simulink model "youhua_1226"  (R2017b)
settings: Solver=ode1  StartTime=0.0  StopTime=Inf  FixedStep=0.0002  RelTol=1e-3
PreLoadFcn:
  | initFun_4P.m
PostLoadFcn:
  | , if any(exist('dsrtsu_mdlpostloadfcn', 'file') == [2, 3, 6]), try dsrtsu_mdlpostloadfcn('Execute', bdroot); catch fprintf('Error in PostLoadFcn (dsrtsu_mdlpostloadfcn) for model "%s":\n %s\n', bdroot, lasterr); end, end,
InitFcn:
  | initFun_4P
undefined symbols (not defined in the file): CMAES_B_initial, CMAES_C_initial, CMAES_chiN_initial, CMAES_counteval_initial, CMAES_D_initial, CMAES_eigeneval_initial, CMAES_invsqrtC_initial, CMAES_pc_initial, CMAES_ps_initial, CMAES_sigma_initial, CMAES_xmean_initial
libraries: rti1202lib_adc_class1 x20, simulink x8, dsparch4 x6, rti1202serlib x4, rti1202lib_dio_class1 x4, dsextras x3, rtiemclib x2, rti1202lib_dac_class1 x1, rtitasklib x1
(part 4 of 6)

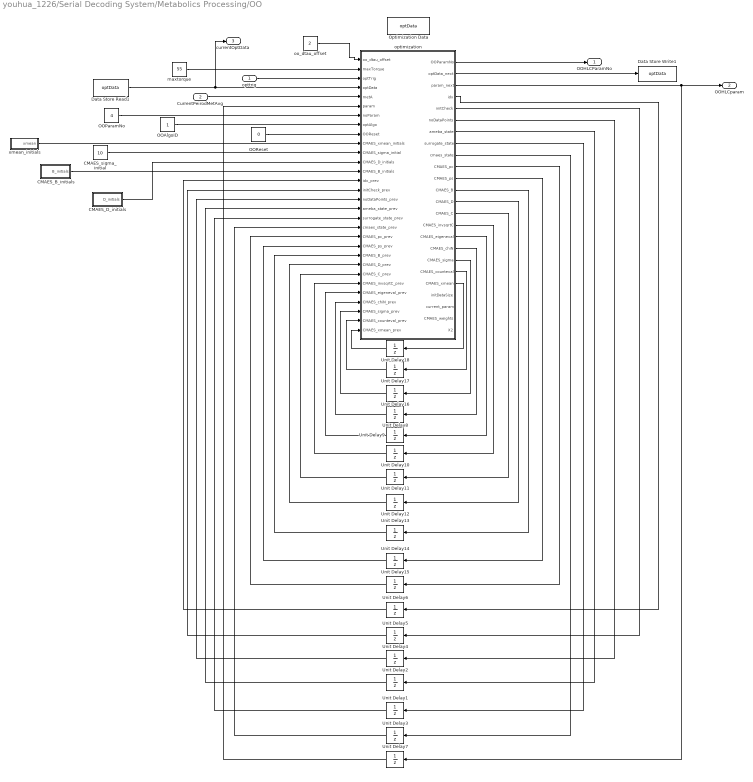
== system youhua_1226/Serial Decoding System/Metabolics Processing/OO ==
  opttrig : Inport
  CurrentPeirodMetAvg : Inport  Port=2
  CMAES_B_initials : Subsystem
  CMAES_D_initials : Subsystem
  CMAES_sigma_initial : Constant  Value=10
  Data Store Read1 : DataStoreRead  DataStoreName=optData
  Data Store Write1 : DataStoreWrite  DataStoreName=optData
  OOAlgoID : Constant
  OOParamNo : Constant  Value=4
  OOReset : Constant  Value=0
  Optimization Data : DataStoreMemory  DataStoreName=optData  ReadBeforeWriteMsg=warning  WriteAfterWriteMsg=warning  WriteAfterReadMsg=warning  InitialValue=zeros(8,5)  ShowAdditionalParam=off
  Unit Delay{1..6} (6 alike) : UnitDelay  SampleTime=-1
  Unit Delay10 : UnitDelay  InitialCondition=CMAES_invsqrtC_initial  SampleTime=-1
  Unit Delay11 : UnitDelay  InitialCondition=CMAES_C_initial  SampleTime=-1
  Unit Delay12 : UnitDelay  InitialCondition=CMAES_D_initial  SampleTime=-1
  Unit Delay13 : UnitDelay  InitialCondition=CMAES_B_initial  SampleTime=-1
  Unit Delay14 : UnitDelay  InitialCondition=CMAES_ps_initial  SampleTime=-1
  Unit Delay15 : UnitDelay  InitialCondition=CMAES_pc_initial  SampleTime=-1
  Unit Delay16 : UnitDelay  InitialCondition=CMAES_sigma_initial  SampleTime=-1
  Unit Delay17 : UnitDelay  InitialCondition=CMAES_counteval_initial  SampleTime=-1
  Unit Delay18 : UnitDelay  InitialCondition=CMAES_xmean_initial  SampleTime=-1
  Unit Delay7 : UnitDelay  InitialCondition=zeros(4,1)  SampleTime=-1
  Unit Delay8 : UnitDelay  InitialCondition=CMAES_chiN_initial  SampleTime=-1
  Unit Delay9 : UnitDelay  InitialCondition=CMAES_eigeneval_initial  SampleTime=-1
  maxtorque : Constant  Value=55
  oo_dtau_offset : Constant  Value=2
  optimization : MATLAB Function  TreatAsAtomicUnit=on
  xmean_initials : Subsystem
  OOHLCParamNo : Outport
  OOHLCparam : Outport  Port=2
  currentOptData : Outport  Port=3
  wires:
  Data Store Read1/1 -> optimization/4(optData), currentOptData/1
  OOAlgoID/1 -> optimization/8(optAlgo)
  CurrentPeirodMetAvg/1 -> optimization/5(metA)
  optimization/3(param_next) -> Unit Delay7/1, OOHLCparam/1
  optimization/2(optData_next) -> Data Store Write1/1
  optimization/1(OOParamNo) -> OOHLCParamNo/1
  OOParamNo/1 -> optimization/7(noParam)
  optimization/4(idx) -> Unit Delay6/1
  Unit Delay7/1 -> optimization/6(param)
  Unit Delay6/1 -> optimization/14(idx_prev)
  OOReset/1 -> optimization/9(OOReset)
  optimization/5(initCheck) -> Unit Delay5/1
  Unit Delay5/1 -> optimization/15(initCheck_prev)
  optimization/6(noDataPoints) -> Unit Delay4/1
  Unit Delay4/1 -> optimization/16(noDataPoints_prev)
  Unit Delay2/1 -> optimization/17(ameba_state_prev)
  optimization/7(ameba_state) -> Unit Delay2/1
  optimization/8(surrogate_state) -> Unit Delay1/1
  Unit Delay1/1 -> optimization/18(surrogate_state_prev)
  optimization/9(cmaes_state) -> Unit Delay3/1
  Unit Delay3/1 -> optimization/19(cmaes_state_prev)
  optimization/17(CMAES_chiN) -> Unit Delay8/1
  Unit Delay8/1 -> optimization/27(CMAES_chiN_prev)
  optimization/16(CMAES_eigeneval) -> Unit Delay9/1
  Unit Delay9/1 -> optimization/26(CMAES_eigeneval_prev)
  optimization/15(CMAES_invsqrtC) -> Unit Delay10/1
  Unit Delay10/1 -> optimization/25(CMAES_invsqrtC_prev)
  optimization/14(CMAES_C) -> Unit Delay11/1
  Unit Delay11/1 -> optimization/24(CMAES_C_prev)
  optimization/13(CMAES_D) -> Unit Delay12/1
  optimization/12(CMAES_B) -> Unit Delay13/1
  optimization/11(CMAES_ps) -> Unit Delay14/1
  optimization/10(CMAES_pc) -> Unit Delay15/1
  Unit Delay12/1 -> optimization/23(CMAES_D_prev)
  Unit Delay13/1 -> optimization/22(CMAES_B_prev)
  Unit Delay14/1 -> optimization/21(CMAES_ps_prev)
  Unit Delay15/1 -> optimization/20(CMAES_pc_prev)
  optimization/18(CMAES_sigma) -> Unit Delay16/1
  Unit Delay16/1 -> optimization/28(CMAES_sigma_prev)
  optimization/19(CMAES_counteval) -> Unit Delay17/1
  Unit Delay17/1 -> optimization/29(CMAES_counteval_prev)
  optimization/20(CMAES_xmean) -> Unit Delay18/1
  Unit Delay18/1 -> optimization/30(CMAES_xmean_prev)
  opttrig/1 -> optimization/3(optTrig)
  CMAES_sigma_initial/1 -> optimization/11(CMAES_sigma_initial)
  xmean_initials/1(xmean) -> optimization/10(CMAES_xmean_initials)
  CMAES_D_initials/1(D_initials) -> optimization/12(CMAES_D_initials)
  maxtorque/1 -> optimization/2(maxTorque)
  CMAES_B_initials/1(B_initials) -> optimization/13(CMAES_B_initials)
  oo_dtau_offset/1 -> optimization/1(oo_dtau_offset)

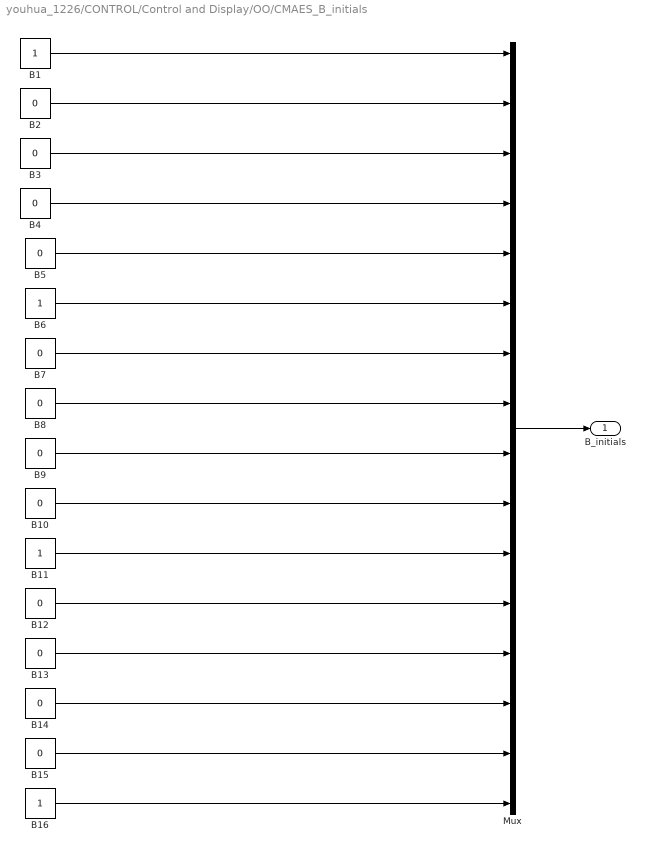
== system youhua_1226/CONTROL/Control and Display/OO/CMAES_B_initials ==
  B{1,6,11,16} (4 alike) : Constant
  B{2..5,7..10,12..15} (12 alike) : Constant  Value=0
  Mux : Mux  Inputs=16
  B_initials : Outport
  wires:
  B1/1 -> Mux/1
  B3/1 -> Mux/3
  B4/1 -> Mux/4
  B2/1 -> Mux/2
  Mux/1 -> B_initials/1
  B5/1 -> Mux/5
  B7/1 -> Mux/7
  B8/1 -> Mux/8
  B6/1 -> Mux/6
  B9/1 -> Mux/9
  B11/1 -> Mux/11
  B12/1 -> Mux/12
  B10/1 -> Mux/10
  B13/1 -> Mux/13
  B15/1 -> Mux/15
  B16/1 -> Mux/16
  B14/1 -> Mux/14

== system youhua_1226/CONTROL/Control and Display/OO/CMAES_D_initials ==
  D{1..4} (4 alike) : Constant
  Mux : Mux
  D_initials : Outport
  wires:
  D1/1 -> Mux/1
  D3/1 -> Mux/3
  D4/1 -> Mux/4
  D2/1 -> Mux/2
  Mux/1 -> D_initials/1

== system youhua_1226/CONTROL/Control and Display/OO/xmean_initials ==
  Mux : Mux
  xmean1 : Constant  Value=25
  xmean2 : Constant  Value=90
  xmean3 : Constant  Value=25
  xmean4 : Constant  Value=20
  xmean : Outport
  wires:
  xmean1/1 -> Mux/1
  xmean3/1 -> Mux/3
  xmean4/1 -> Mux/4
  xmean2/1 -> Mux/2
  Mux/1 -> xmean/1

== system youhua_1226/CONTROL/Control and Display/learning data read/filtered step data read ==
  indices : Inport
  comm delay cycle : Inport  Port=2
  learningMode : Inport  Port=3
  "   " : SignalSpecification  Dimensions=3
  "       currentstepdata" : DataStoreRead  DataStoreName=filteredStepData
  Step Data Access : MATLAB Function  TreatAsAtomicUnit=on
  oldD : Outport
  wires:
  "       currentstepdata"/1 -> Step Data Access/2(oldSD)
  Step Data Access/1(oldD) -> "   "/1
  indices/1 -> Step Data Access/1(indices)
  "   "/1 -> oldD/1
  comm delay cycle/1 -> Step Data Access/3(CommDelayCycle)
  learningMode/1 -> Step Data Access/4(learningMode)

== system youhua_1226/CONTROL/Control and Display/learning data write/filtered step data write ==
  indices : Inport
  filteredstepdata : Inport  Port=2
  learningMode : Inport  Port=3
  BT Reset3 : Constant  Value=0
  MATLAB Function2 : MATLAB Function  TreatAsAtomicUnit=on
  filtered data store read : DataStoreRead  DataStoreName=filteredStepData
  filtered data store write : DataStoreWrite  DataStoreName=filteredStepData
  wires:
  filtered data store read/1 -> MATLAB Function2/4(filtered_step_data_in)
  MATLAB Function2/1(filtered_step_data_out) -> filtered data store write/1
  BT Reset3/1 -> MATLAB Function2/1(bt_reset3)
  indices/1 -> MATLAB Function2/2(indices)
  filteredstepdata/1 -> MATLAB Function2/3(filtered_step_data)
  learningMode/1 -> MATLAB Function2/5(learningMode)

== system youhua_1226/CONTROL/Control and Display/time derivatives /get ddot torque ==
  data : Inport
  Butterworth Filter (low 100Hz) : DiscreteFilter  Numerator="[0.0181    0.0543    0.0543    0.0181]"  Denominator="[ 1.0000   -1.7600    1.1829   -0.2781]"
  Discrete Derivative : simulink/Discrete/Discrete Derivative  gainval=1.0  ICPrevScaledInput=0.0  InputProcessing=Inherited  OutMin=[]  OutMax=[]  OutDataType=fixdt(1, 16)  OutScaling=2^-10  DoSatur=off
  dotdata : Outport
  wires:
  Discrete Derivative/1 -> Butterworth Filter (low 100Hz)/1
  data/1 -> Discrete Derivative/1
  Butterworth Filter (low 100Hz)/1 -> dotdata/1

== system youhua_1226/CONTROL/Control and Display/time derivatives /get desired torque  ==
  data : Inport
  Butterworth Filter (low 100Hz) : DiscreteFilter  Numerator="[0.0181    0.0543    0.0543    0.0181]"  Denominator="[ 1.0000   -1.7600    1.1829   -0.2781]"
  Discrete Derivative : simulink/Discrete/Discrete Derivative  gainval=1.0  ICPrevScaledInput=0.0  InputProcessing=Inherited  OutMin=[]  OutMax=[]  OutDataType=fixdt(1, 16)  OutScaling=2^-10  DoSatur=off
  dotdata : Outport
  wires:
  Discrete Derivative/1 -> Butterworth Filter (low 100Hz)/1
  data/1 -> Discrete Derivative/1
  Butterworth Filter (low 100Hz)/1 -> dotdata/1

== system youhua_1226/CONTROL/Control and Display/time derivatives /get desired torque 1 ==
  data : Inport
  Butterworth Filter (low 100Hz) : DiscreteFilter  Numerator="[0.0181    0.0543    0.0543    0.0181]"  Denominator="[ 1.0000   -1.7600    1.1829   -0.2781]"
  Discrete Derivative : simulink/Discrete/Discrete Derivative  gainval=1.0  ICPrevScaledInput=0.0  InputProcessing=Inherited  OutMin=[]  OutMax=[]  OutDataType=fixdt(1, 16)  OutScaling=2^-10  DoSatur=off
  dotdata : Outport
  wires:
  Discrete Derivative/1 -> Butterworth Filter (low 100Hz)/1
  data/1 -> Discrete Derivative/1
  Butterworth Filter (low 100Hz)/1 -> dotdata/1

== system youhua_1226/CONTROL/Control and Display/time derivatives /get desired torque 2 ==
  data : Inport
  Butterworth Filter (low 100Hz) : DiscreteFilter  Numerator="[0.0181    0.0543    0.0543    0.0181]"  Denominator="[ 1.0000   -1.7600    1.1829   -0.2781]"
  Discrete Derivative : simulink/Discrete/Discrete Derivative  gainval=1.0  ICPrevScaledInput=0.0  InputProcessing=Inherited  OutMin=[]  OutMax=[]  OutDataType=fixdt(1, 16)  OutScaling=2^-10  DoSatur=off
  dotdata : Outport
  wires:
  Discrete Derivative/1 -> Butterworth Filter (low 100Hz)/1
  data/1 -> Discrete Derivative/1
  Butterworth Filter (low 100Hz)/1 -> dotdata/1

== system youhua_1226/RTI Data/RTI Data Store/RTI Data Store/RTI Data Store ==
  RTI Data Store : Subsystem  mask(RTI_DATA_STORE){}
      mask help:
      | RTI Data Store Block. This block is used by RTI to store internal model dependent data. Deleting this block will result in data loss.
      |
      | NEVER DELETE, COPY, OR MODIFY THIS BLOCK!
      mask Help:
      | RTI Data Store Block. This block is used by RTI to store internal model dependent data. Deleting this block will result in data loss.
      | 
      | NEVER DELETE, COPY, OR MODIFY THIS BLOCK!
      mask Display: text(0.5, 0.5, ' ', 'HorizontalAlignment', 'center');

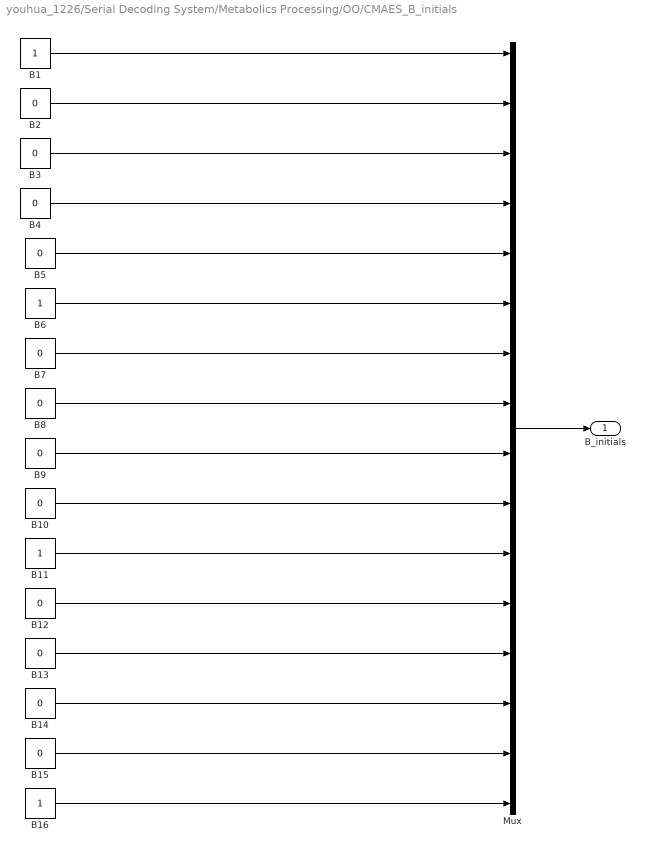
== system youhua_1226/Serial Decoding System/Metabolics Processing/OO/CMAES_B_initials ==
  B{1,6,11,16} (4 alike) : Constant
  B{2..5,7..10,12..15} (12 alike) : Constant  Value=0
  Mux : Mux  Inputs=16
  B_initials : Outport
  wires:
  B1/1 -> Mux/1
  B3/1 -> Mux/3
  B4/1 -> Mux/4
  B2/1 -> Mux/2
  Mux/1 -> B_initials/1
  B5/1 -> Mux/5
  B7/1 -> Mux/7
  B8/1 -> Mux/8
  B6/1 -> Mux/6
  B9/1 -> Mux/9
  B11/1 -> Mux/11
  B12/1 -> Mux/12
  B10/1 -> Mux/10
  B13/1 -> Mux/13
  B15/1 -> Mux/15
  B16/1 -> Mux/16
  B14/1 -> Mux/14

== system youhua_1226/Serial Decoding System/Metabolics Processing/OO/CMAES_D_initials ==
  D{1..4} (4 alike) : Constant
  Mux : Mux
  D_initials : Outport
  wires:
  D1/1 -> Mux/1
  D3/1 -> Mux/3
  D4/1 -> Mux/4
  D2/1 -> Mux/2
  Mux/1 -> D_initials/1

== system youhua_1226/Serial Decoding System/Metabolics Processing/OO/xmean_initials ==
  Mux : Mux
  xmean1 : Constant  Value=25
  xmean2 : Constant  Value=90
  xmean3 : Constant  Value=25
  xmean4 : Constant  Value=20
  xmean : Outport
  wires:
  xmean1/1 -> Mux/1
  xmean3/1 -> Mux/3
  xmean4/1 -> Mux/4
  xmean2/1 -> Mux/2
  Mux/1 -> xmean/1

== system youhua_1226/RTI Data/RTI Data Store/RTI Data Store/RTI Data Store/RTI Data Store ==

== matlab function youhua_1226/Sensor Data Conversion/bit data processing ==
  data: bit_data input; heel_switch output
function heel_switch = fcn(bit_data)

heel_switch = bit_data(1);

% heel_switch = ~heel_switch;

return;

== matlab function youhua_1226/Sensor Data Conversion/analog data processing ==
  data: adc_data input; ankle_pos output; enc_pos input; load_vol_gain input; load_vol_offset input; CPR_ankle input; CPR_motor input; analog_enc_max input; analog_enc_min input; BT_RESET_TORQUE input; force_input0_prev input; motor_pos output; load_cell_vol output; force_input output; EMG1_vol output; force_input0_next output; fzright_raw output; fzleft_raw output
function [ankle_pos, motor_pos, load_cell_vol, force_input, EMG1_vol, force_input0_next,...
    fzright_raw, fzleft_raw]=fcn(adc_data,enc_pos,...
    load_vol_gain,load_vol_offset, CPR_ankle, CPR_motor, analog_enc_max,...
    analog_enc_min, BT_RESET_TORQUE, force_input0_prev)
%#eml
ankle_pos = enc_pos(1)*360/CPR_ankle;
%% analog encoder
% ankle_pos = (adc_data(17)-analog_enc_min)*360/(analog_enc_max-analog_enc_min);
% if ankle_pos >180
%     ankle_pos = ankle_pos - 360;
% end;
% ankle_pos = - ankle_pos;
%%
motor_pos = enc_pos(2)*360/CPR_motor;%CPR_motor = 1250光栅参数
%load_cell_vol 放大器输出电压*10的数值
load_cell_vol = adc_data(6);
%电压力矩转换 load_vol_gain = 9.9206 load_vol_offset = 11.4484；
%force_input_raw  =   load_cell_vol*load_vol_gain/5.5 + load_vol_offset;
force_input_raw  =   load_cell_vol*load_vol_gain + load_vol_offset;
% force_input_raw = max(force_input_raw, 0);
% 力矩调零 BT_RESET_TORQUE （力矩调零按钮）
if BT_RESET_TORQUE ==1
    force_input0_next = force_input_raw;
    
else
    force_input0_next = force_input0_prev;
    
end

force_input = force_input_raw - force_input0_next;
%未知
EMG1_vol = adc_data(5);

fzright_raw = adc_data(11);
fzleft_raw = adc_data(15);

return

== matlab function youhua_1226/CONTROL/Control and Display/State Operation ==
  data: tmp1 output; tmp2 output; reset_torque_swing input; max_desired_torque input; max_motor_pos input; max_motor_pos_inv input; desired_motor_velocity output; current_state_input input; analog_inputs input; user_inputs input; digital_inputs input; state_variables0 input; time input; time_derivatives input; filtered_lrn_data input; CusHLCInputs input; serial_data input; opt_data input; desired_vel_prev input; tau_offset_prev input; state_variables output; current_step_data output; Params output; measured_torque output; ankle_pos output; motor_pos output; desired_torque output; tau_offset output
function [tmp1, tmp2, desired_motor_velocity, state_variables, current_step_data,Params,measured_torque,ankle_pos,motor_pos,desired_torque, tau_offset]  =...
    fcn(reset_torque_swing, max_desired_torque,max_motor_pos,max_motor_pos_inv,current_state_input, analog_inputs,user_inputs, digital_inputs,...
    state_variables0, time,  time_derivatives, filtered_lrn_data,...
    CusHLCInputs,serial_data, opt_data, desired_vel_prev,tau_offset_prev)


% defination
%State definitions
idle_state	=	0;
calibration_state	=   1;
stance_state   =   2;
swing_state     =   3;
step_state  =   4;
slack_state = 5;
pos_track_state = 6;
%   Constants
gearRatio = 5;



maximum_motor_velocity = 90*360; %maximum allowable motor velocity (deg/s)


current_state = current_state_input(1);
stop_pos = current_state_input(2);
slack_pos = current_state_input(3);
stance_end_pos = current_state_input(4);
flag_d_p = current_state_input(6);
dorsi_end_pos = current_state_input(15);
last_stride_time = current_state_input(13);


% vo2 = serial_data(1);
% vco2 = serial_data(2);
% metE = serial_data(3);
%
% metA = opt_data(1);
HLCParamNo = opt_data(2);
HLCParam = opt_data(3:HLCParamNo+2);
Params = opt_data(3:end);



% load_pivot_distance = 0;
% load_angle = 0;

% state variables initialization
zero_ankle_pos_prev =  state_variables0(1);
zero_motor_pos_prev = state_variables0(2);
ankle_pos_prev = state_variables0(3);
motor_pos_prev = state_variables0(4);
desired_torque_prev = state_variables0(5);
measured_torque_prev = state_variables0(6);
measured_force_prev = state_variables0(7);
load_angle_prev = state_variables0(8);
load_pivot_distance_prev = state_variables0(9);
delta_motor_pos_prev = state_variables0(10);
slack_motor_pos_prev = state_variables0(11);
torque_error_prev = state_variables0(12);
Kp_prev = state_variables0(13);
ankle_vel_prev = state_variables0(14);
motor_vel_prev = state_variables0(15);
motor_acc_prev = state_variables0(16);
Kd_prev = state_variables0(17);
Ki_prev = state_variables0(18);
Controller_prev = state_variables0(19);
Kc_prev = state_variables0(20);
time_prev = state_variables0(21);
state_prev = state_variables0(22);
state_start_time_prev = state_variables0(23);
curve_id_prev = state_variables0(24);
Kpp_prev = state_variables0(25);
accumulated_torque_error_prev = state_variables0(26);
desired_motor_pos_prev = state_variables0(27);
walk_control_mode_prev = state_variables0(28);
prev_step_accumulated_error_prev = state_variables0(29);
curr_step_accumulated_error_prev = state_variables0(30);
learning_control_input_prev = state_variables0(31);

learning_control_input2_prev = state_variables0(32);
Kp2_prev = state_variables0(33);
Kl_prev = state_variables0(34);
Kl2_prev = state_variables0(35);
gamma_prev = state_variables0(37);
Lce_prev = state_variables0(38);
Lmtu_prev = state_variables0(39);
FL_prev = state_variables0(40);
Fpe_prev = state_variables0(41);
ACT_prev = state_variables0(42);
STIM_Prev = state_variables0(43);
Fmtu_prev = state_variables0(44);
Lcedot_prev = state_variables0(45);
learned_value_prev = state_variables0(46);
learned_avg_prev = state_variables0(47);
accumulated_pos_error_prev = state_variables0(48);
gamma1_prev = state_variables0(49);
gamma2_prev = state_variables0(50);
gamma3_prev = state_variables0(51);
gamma4_prev = state_variables0(52);
gamma_v_prev = [gamma1_prev;gamma2_prev;gamma3_prev;gamma4_prev];




%% if no updation, use the old ones
zero_motor_pos = zero_motor_pos_prev; %if no new zero points set, keep old ones
zero_ankle_pos = zero_ankle_pos_prev;
ankle_pos = ankle_pos_prev;
motor_pos = motor_pos_prev;
desired_torque = desired_torque_prev;
measured_torque = measured_torque_prev;
measured_force = measured_force_prev;
load_angle = load_angle_prev;
load_pivot_distance = load_pivot_distance_prev;
delta_motor_pos = delta_motor_pos_prev;
slack_motor_pos = slack_motor_pos_prev;
torque_error = torque_error_prev;
Kp = Kp_prev;
ankle_vel = ankle_vel_prev;
motor_vel = motor_vel_prev;
motor_acc = motor_acc_prev;
Kd = Kd_prev;
Ki = Ki_prev;
Controller = Controller_prev;
Kc = Kc_prev;
current_time = time_prev;
state = state_prev;
state_start_time = state_start_time_prev;
curve_id = curve_id_prev;
Kpp = Kpp_prev;
accumulated_torque_error = accumulated_torque_error_prev;
desired_motor_pos = desired_motor_pos_prev;
walk_control_mode  = walk_control_mode_prev;
prev_step_accumulated_error=prev_step_accumulated_error_prev;
curr_step_accumulated_error=curr_step_accumulated_error_prev;
learning_control_input = learning_control_input_prev;
learning_control_input2 = learning_control_input2_prev;
Kp2 = Kp2_prev;
Kl = Kl_prev;
Kl2 = Kl2_prev;
gamma = gamma_prev;

Lce = Lce_prev;
Lmtu = Lmtu_prev;
FL = FL_prev;
Fpe = Fpe_prev;
ACT = ACT_prev ;
STIM = STIM_Prev ;
Fmtu = Fmtu_prev ;
Lcedot = Lcedot_prev;
learned_value  = learned_value_prev;
learned_avg = learned_avg_prev;
accumulated_pos_error = accumulated_pos_error_prev;
gamma1 = gamma1_prev;
gamma2 = gamma2_prev;
gamma3 = gamma3_prev;
gamma4 = gamma4_prev;
gamma_v = gamma_v_prev;
state_variables = state_variables0;

% learned_avg = step_avg_data;


tau_offset = tau_offset_prev;







% foot_switch     =   digital_inputs(1);
load_cell_vol = analog_inputs(3);
measured_ankle_pos = analog_inputs(1);
measured_motor_pos = analog_inputs(2);
measured_force = analog_inputs(4);
ankle_vel = analog_inputs(5);
motor_vel = analog_inputs(6);
force_vel = analog_inputs(7);
motor_acc = analog_inputs(8);
EMG1_vol = analog_inputs(9);


Kp = user_inputs(1);
load_distance_1 = user_inputs(2); % in inches
load_distance_2 = user_inputs(3); % in inches
load_ankle_offset = user_inputs(4); % in degrees
delta_t_motor = user_inputs(6);
user_motor_speed = user_inputs(7);
desired_torque = user_inputs(8);
Kd = user_inputs(9);
Ki = user_inputs(10);
Controller = user_inputs(11);
Kc = user_inputs(12);
system_delay = user_inputs(13)/1000;
curve_id = user_inputs(14);
Kpp = user_inputs(15);
sine_freq = user_inputs(16);
Kt = user_inputs(17);
stance_motor_offset = user_inputs(18);
stance_motor_speed = user_inputs(19);
swing_motor_slack = user_inputs(20);
walk_control_mode = user_inputs(21);
slack_length = user_inputs(22);
desired_torque_magnitude = user_inputs(23);
Kl = user_inputs(24);
Kl2 = user_inputs(25);
x1 = user_inputs(26);
y1 = user_inputs(27);
xinit = user_inputs(28);
xturn = user_inputs(29);
yturn = user_inputs(30);
Cw = user_inputs(31);
Kpa= user_inputs(32);
load_pivot_distance = user_inputs(33);
torque_offset = user_inputs(34);
K_curve = user_inputs(35);
K_amp = user_inputs(36);
K_s = user_inputs(37);
L_adpt = user_inputs(38);


%% parameters of NMM

est_stride_time = user_inputs(54);
EMG_OFFSET = user_inputs(58);


%% eroror dependant p parames
ed_p_taumax = user_inputs(60);
ed_p_taustep = user_inputs(61);
%%
comm_delay_cycle = user_inputs(62);
isModiAdded = user_inputs(63);
%% position tracking performance test
Pos_Kd = user_inputs(64);
Pos_Ki = user_inputs(65);
%%
alpha = user_inputs (66);

%% passivity
lambda = user_inputs(67);
%%
isPosPID = user_inputs(68);
%% for learning control threshold

lrn_tau_err_threshold = user_inputs(69);
lrn_shrink_rate = user_inputs(70);

K_swing_follow = user_inputs(72);
r_motor_shaft = user_inputs(73);

%% for ankle-based curve

maxPlanter = user_inputs(74);
xadjust_ref = user_inputs(75);
yadjust_ref = user_inputs(76);


curve_k2 = user_inputs(78);
pos_traj_mode = user_inputs(79);
pos_des_1 = user_inputs(80);
pos_des_2 = user_inputs(81);

Kp_early_swing = user_inputs(82);

oo_dtau_offset = user_inputs(83);


%% for learning control
previous_filtered_torque_error = filtered_lrn_data(1); %torque error of same index of last step

previous_learning_control_input = filtered_lrn_data(2);
predicted_learning_control_input = filtered_lrn_data(3);

% torque_error = previous_filtered_torque_error;
current_learning_control_input = previous_learning_control_input;
current_step_data = [torque_error; current_learning_control_input; previous_filtered_torque_error];

%%
% 脚踝与电机编码器角度调零
motor_pos = measured_motor_pos - zero_motor_pos;
ankle_pos = measured_ankle_pos - zero_ankle_pos;


% load_input      =   load_cell_vol*load_vol_gain + load_vol_offset;
% if measured_force < 0
%     measured_force = 0;
% end;
load_angle = load_ankle_offset - ankle_pos;
% load_pivot_distance = load_distance_1*load_distance_2*sin(load_angle*pi/180)/sqrt(load_distance_1^2+load_distance_2^2+2*load_distance_1*load_distance_2*cos(load_angle*pi/180));
% load_pivot_distance = 3.7808;
% 1`111111111111111`1
% measured_torque =   measured_force*load_pivot_distance-torque_offset;
% 原本是在此处由力转成力矩，由于之前force_input已经直接转化为力矩，所以这里直接用 measured_torque =   measured_force;
% measured_torque = max(0, measured_torque);
measured_torque =   measured_force;


% desired_torque  =   20;

%%%%%%%%%%%%%%%%%%% state variables update%%%%%%%%%%%%%%%%%%%%%%%%%%%%%%%%%
current_time = time;
state = current_state;

%--------------
tmp1 = state;
tmp2 = state_prev;
%--------------
if state~= state_prev
    state_start_time = current_time;
    accumulated_torque_error = 0;
    accumulated_pos_error = 0;
    gamma1_prev = 0;
    gamma2_prev = 0;
    gamma3_prev = 0;
    gamma4_prev = 0;
    if state == stance_state
        prev_step_accumulated_error = curr_step_accumulated_error;
        curr_step_accumulated_error = 0;
        learning_control_input = 0;
        
    end;
    if state == idle_state
        prev_step_accumulated_error = 0;
        curr_step_accumulated_error = 0;
        learning_control_input = 0;
        Kp2 = 0;
        learning_control_input2 =0;
    end;
    if state == swing_state && state_prev ~= stance_state % start of walk
        %         gamma1 = 0;
        %         gamma2 = 0;
        %         gamma3 = 0;
        %         gamma4 = 0;
        %         gamma_v = [0 0 0 0]';
        gamma1_prev = 0;
        gamma2_prev = 0;
        gamma3_prev = 0;
        gamma4_prev = 0;
        %         gamma_v_prev  = [ 0 0 0 0]';
    end
end;

%%%%%%%%%%% variables update finished
if flag_d_p==0
    Cw=0;
end;



%生成期望力矩曲线；curve_id：期望曲线类型  last_stride_time: 1 or 1.5  
%CusHLCInputs 力矩曲线的四参数 ：peak_torque peak_time rise_time drop_time
%oo_dtau_offset
%HLCParam
%xinit
desired_torque = torque_curve(current_time, state_start_time,...
    current_state, curve_id,...
    desired_torque_magnitude,...
    last_stride_time, HLCParam, ankle_pos, xinit,K_curve, CusHLCInputs, oo_dtau_offset);
%期望力矩不能超过120（单位不一样可能需要调整）
desired_torque = min(desired_torque, max_desired_torque);
if state==stance_state
    torque_error = measured_torque-desired_torque;
else
    torque_error = 0;
end

%% for learning with filtered torque
filtered_torque_error = previous_filtered_torque_error*(1-alpha) + alpha*torque_error;
%%
accumulated_torque_error = torque_error + accumulated_torque_error;
accumulated_pos_error = accumulated_pos_error_prev + desired_motor_pos - motor_pos;
if state == stance_state
    curr_step_accumulated_error = curr_step_accumulated_error + torque_error*0.002;
end


%% time derivatives
dot_desired_torque = time_derivatives(1);
ddot_desired_torque = time_derivatives(2);
dot_desired_motor_pos = time_derivatives(3);
dot_measured_torque = time_derivatives(4);

%% passivity based control 存疑
% s = lambda*torque_error + dot_measured_torque-dot_desired_torque;
% Y = [measured_torque; dot_desired_torque-lambda*torque_error; ddot_desired_torque-lambda*(dot_measured_torque - dot_desired_torque); ankle_vel]';
s = lambda*torque_error -motor_vel;
Y = [measured_torque; -lambda*torque_error; lambda*motor_vel; ankle_vel]';
gamma_v_prev = [gamma1_prev;gamma2_prev;gamma3_prev;gamma4_prev];
gamma_v = gamma_v_prev + delta_t_motor*(-L_adpt*Y'*s);
% Y = 0
% gamma_v = [ 0 0 0 0]';
gamma1 = gamma_v(1);
gamma2 = gamma_v(2);
gamma3 = gamma_v(3);
gamma4 = gamma_v(4);


% 存疑 
motor_pos_modifer = isModiAdded*motor_vel*comm_delay_cycle*0.002*gearRatio/delta_t_motor;
posTrack_modifier = isPosPID*(-Pos_Kd*(dot_desired_motor_pos - motor_vel)*gearRatio-Pos_Ki*gearRatio*accumulated_pos_error);


% 力矩调零 由于reset_torque_swing = 0 所以暂时没用到 tau_offset = 0
if reset_torque_swing ==1
    if current_state == swing_state
        if (current_time - state_start_time)> 0.15 && (current_time - state_start_time)< 0.2
            tau_offset = measured_torque;
        end
    end
end

if reset_torque_swing ==2
tau_offset = 0;
end

measured_torque = measured_torque - tau_offset; % dynamic resetting 

switch current_state
    case idle_state
        %               desired_motor_velocity = -(motor_pos-motor_pos_prev)/delta_t_motor;
        if stop_pos == 0 %stop_pos = motor_pos_prev
            desired_motor_velocity = 0;
        else
            delta_motor_pos = (stop_pos -motor_pos);
            desired_motor_pos = stop_pos;
            desired_motor_velocity = -(delta_motor_pos*gearRatio/delta_t_motor);
        end
    % 调整脚踝与电机编码器角度为零的状态，记录当前编码器角度，下一个采样时做差调零
    case calibration_state 
        zero_motor_pos = measured_motor_pos;
        zero_ankle_pos = measured_ankle_pos;
        slack_motor_pos = measured_motor_pos;
        desired_motor_velocity = user_motor_speed;
        %       desired_torque = torque_curve(current_time, state_start_time, Controller, current_state, curve_id, sine_freq, ankle_pos, Kt);
    % 未知    
    case step_state
        switch Controller
            
            otherwise
                desired_motor_velocity = 0;
        end
        
    case stance_state
        %delta_t_motor的值可能需要调整，当前为0.05 会使控制电压过大
        switch walk_control_mode
            case 1 % torque control % PAPER CONTROLLER 1 & 2, Kpp = zero, nonzero 力矩控制 Kpp = 0 Ki = 0
                delta_motor_pos = Kpp*(-ankle_pos*load_pivot_distance/r_motor_shaft - desired_torque/Kc-motor_pos)-Kp*(desired_torque-measured_torque)-Kd*motor_vel-Ki*(-accumulated_torque_error);
                desired_motor_pos = delta_motor_pos + motor_pos;
                desired_motor_velocity = -delta_motor_pos*gearRatio/delta_t_motor;
                %测试时电机旋转方向错误，将负号去掉；
                %新：desired_motor_vrlocity = 4000 的问题可能因为Kd*motor_vel
                %新：环路成为一个正反馈，所以把第三行负号加上
                %加上motor_pos_modifer+posTrack_modifier这两项会使控制电压到达阈值2000（暂不清楚原因）
                %这两项的值当前都为 0 ？？
%               desired_motor_velocity = -(delta_motor_pos*gearRatio/delta_t_motor)+motor_pos_modifer + posTrack_modifier;
                
                %             case 6 %damping on relative speed instead of absolute speedC
                %                 desired_motor_pos = -ankle_pos*load_pivot_distance/r_motor_shaft*K_swing_follow+swing_motor_slack;
                %                 delta_motor_pos =(desired_motor_pos-motor_pos);
                %                 desired_motor_velocity = -(delta_motor_pos*gearRatio/delta_t_motor);
            case 9 % passive walking
                desired_motor_pos = 0;
                desired_motor_velocity = -((desired_motor_pos-motor_pos)*gearRatio/delta_t_motor);
                %             case 17 %passivity based controller
                %                 delta_motor_pos  = -Kp*(desired_torque-measured_torque)-K_s*(-s)-Y*gamma_v;
                %                 desired_motor_pos = delta_motor_pos + motor_pos;
                %                 desired_motor_velocity = -((desired_motor_pos-motor_pos)*gearRatio/delta_t_motor)+motor_pos_modifer + posTrack_modifier;
                %             case 18 % PAPER CONTROLLER 4 position based stiffness, saturated at 100 torque error
                %                 max_cnt = ceil(ed_p_taumax/ed_p_taustep);
                %                 temp_cnt = ceil(abs(desired_torque-measured_torque)/ed_p_taustep);
                %                 Kpc = Kp*temp_cnt/max_cnt;
                %                 %                 Kpc = Kp*(desired_torque-measured_torque)/100;
                %                 Kpc = min(Kp, Kpc);
                %                 delta_motor_pos = Kpp*(-ankle_pos*load_pivot_distance/r_motor_shaft - desired_torque/Kc-motor_pos)-Kpc*(desired_torque-measured_torque)-Kd*motor_vel-Ki*(-accumulated_torque_error);
                %                 desired_motor_pos = delta_motor_pos + motor_pos;
                %                 desired_motor_velocity = -(delta_motor_pos*gearRatio/delta_t_motor)+motor_pos_modifer + posTrack_modifier;
                %             case 20 % paper controller 6, real-time learning control, kate's method, to be tested
                %                 delta_motor_pos = Kpp*(-ankle_pos*load_pivot_distance/r_motor_shaft - desired_torque/Kc-motor_pos)-Kp*(desired_torque-measured_torque-torque_error_prev)-Kd*motor_vel-Ki*(-accumulated_torque_error);
                %                 desired_motor_velocity = -(delta_motor_pos*gearRatio/delta_t_motor)+motor_pos_modifer + posTrack_modifier;
            case 31 % learning2, with shrink
                current_learning_control_input = previous_learning_control_input*lrn_shrink_rate - Kl*(-filtered_torque_error);
                learned_value = current_learning_control_input;
                desired_motor_pos = predicted_learning_control_input;
                delta_motor_pos = desired_motor_pos - motor_pos;
                desired_motor_velocity = -((desired_motor_pos-motor_pos)*gearRatio/delta_t_motor)+motor_pos_modifer + posTrack_modifier;
            case 32
                current_learning_control_input = previous_learning_control_input*lrn_shrink_rate - Kl*(-filtered_torque_error);
                learned_value = current_learning_control_input;
                desired_motor_pos= predicted_learning_control_input + Kpp*(-ankle_pos*load_pivot_distance/r_motor_shaft - desired_torque/Kc-motor_pos)-Kp*(desired_torque-measured_torque)-Kd*motor_vel-Ki*(-accumulated_torque_error);
                delta_motor_pos = desired_motor_pos - motor_pos;
                desired_motor_velocity = -(delta_motor_pos*gearRatio/delta_t_motor)+motor_pos_modifer + posTrack_modifier;
            case 33
                current_learning_control_input = previous_learning_control_input*lrn_shrink_rate - Kl*(-filtered_torque_error);
                learned_value = current_learning_control_input;
                delta_motor_pos = predicted_learning_control_input + Kpp*(-ankle_pos*load_pivot_distance/r_motor_shaft - desired_torque/Kc-motor_pos)-Kp*(desired_torque-measured_torque)-Kd*motor_vel-Ki*(-accumulated_torque_error);
                desired_motor_pos = delta_motor_pos + motor_pos;
                desired_motor_velocity = -(delta_motor_pos*gearRatio/delta_t_motor);
            case 34 % 测试模式 可以不连接电机与bowden cable 检验电机转向是否正确
                desired_motor_pos = -ankle_pos*load_pivot_distance/r_motor_shaft*K_swing_follow+swing_motor_slack;%K_swing_follow为0-1之间的常数 原式ankle_pos前有负号，测试时因为转向相反所以去掉
                delta_motor_pos =(desired_motor_pos-motor_pos);
                desired_motor_velocity = -(delta_motor_pos*gearRatio/delta_t_motor);
            otherwise
                desired_motor_velocity = 0;
        end
    case swing_state
%         delta_motor_pos = Kpp*(-ankle_pos*load_pivot_distance/r_motor_shaft - desired_torque/Kc-motor_pos)-Kp*(desired_torque-measured_torque)-Kd*motor_vel-Ki*(-accumulated_torque_error);
%                 desired_motor_pos = delta_motor_pos +motor_pos;
%                 desired_motor_velocity = -delta_motor_pos*gearRatio/delta_t_motor;
        desired_motor_pos = -ankle_pos*load_pivot_distance/r_motor_shaft*K_swing_follow+swing_motor_slack;% 同stance case 34 ankle_pos有修改
%         delta_motor_pos =(desired_motor_pos-motor_pos);
        delta_motor_pos =(desired_motor_pos-motor_pos);
        switch walk_control_mode
            case 34
            desired_motor_velocity = -(delta_motor_pos*gearRatio/delta_t_motor);
            case 9
            desired_motor_velocity = -(delta_motor_pos*gearRatio/delta_t_motor);
            otherwise
                if (current_time -state_start_time)<0.1
                    desired_motor_velocity = -Kp_early_swing*(delta_motor_pos*gearRatio/delta_t_motor);
                else
                desired_motor_velocity = -(delta_motor_pos*gearRatio/delta_t_motor);
                end
        end
            
    % 此两种模式暂时未用到    
    case slack_state
        delta_motor_pos = (slack_pos + slack_length -motor_pos);
        desired_motor_pos = slack_pos;
        desired_motor_velocity = -(delta_motor_pos*gearRatio/delta_t_motor);
    case pos_track_state
        desired_motor_pos = pos_trajectory(current_time, state_start_time, pos_traj_mode, pos_des_1, pos_des_2);
        delta_motor_pos = desired_motor_pos-motor_pos;
        desired_motor_velocity = -(delta_motor_pos*gearRatio/delta_t_motor)-Pos_Kd*(dot_desired_motor_pos - motor_vel)*gearRatio-Pos_Ki*gearRatio*accumulated_pos_error;
    otherwise
        desired_motor_velocity = 0;
end
%电机控制电压的大小限制 -2000~2000 （此值需调整：1.单位不统一 2. motor_controller中模块有改动，mint中代码也有改动，还需调整）
desired_motor_velocity = max(-maximum_motor_velocity, min(desired_motor_velocity, maximum_motor_velocity));
% max_motor_acc = 1*10^(6);
% if (desired_motor_velocity - motor_vel*(-5)) >max_motor_acc*0.002
%     desired_motor_velocity = motor_vel*(-5)+ max_motor_acc*0.002;
% end
% if (desired_motor_velocity - motor_vel*(-5)) <-max_motor_acc*0.002
%     desired_motor_velocity = motor_vel*(-5) - max_motor_acc*0.002;
% end

if motor_pos > max_motor_pos 
    desired_motor_velocity = 0;
end

if motor_pos< -max_motor_pos_inv
    desired_motor_velocity = 0;
end
% Lce = Lce + Lcedot*0.002;
% ACT = ACT+adot*0.002;

state_variables(1) = zero_ankle_pos;
state_variables(2) = zero_motor_pos;
state_variables(3) = ankle_pos;
state_variables(4) = motor_pos;
state_variables(5) = desired_torque;
state_variables(6) = measured_torque;
state_variables(7) = measured_force;
state_variables(8) = load_angle;
state_variables(9) = load_pivot_distance;
state_variables(10) = delta_motor_pos;
state_variables(11) = slack_motor_pos;
state_variables(12) = torque_error;
state_variables(13) = Kp;
state_variables(14) = ankle_vel;
state_variables(15) = motor_vel;
state_variables(16) = motor_acc;
state_variables(17) = Kd;
state_variables(18) = Ki;
state_variables(19) = Controller;
state_variables(20) = Kc;
state_variables(21) = current_time;
state_variables(22) = state;
state_variables(23) = state_start_time;
state_variables(24) = curve_id;
state_variables(25) = Kpp;
state_variables(26) = accumulated_torque_error;
state_variables(27) = desired_motor_pos;
state_variables(28) = walk_control_mode;
state_variables(29) = prev_step_accumulated_error;
state_variables(30) = curr_step_accumulated_error;
state_variables(31) = learning_control_input;
state_variables(32) = learning_control_input2;
state_variables(33) = Kp2;
state_variables(34) = Kl;
state_variables(35) = Kl2;
state_variables(36) = flag_d_p;
state_variables(37) = gamma;
state_variables(38) = Lce;
state_variables(39) = Lmtu;
state_variables(40) = FL;
state_variables(41) = Fpe;
state_variables(42) = ACT;
state_variables(43) = STIM;
state_variables(44) = Fmtu;
state_variables(45) = Lcedot;
state_variables(46) = learned_value;
state_variables(47) = 0;
state_variables(48) = accumulated_pos_error;
state_variables(49) = gamma1;
state_variables(50) = gamma2;
state_variables(51) = gamma3;
state_variables(52) = gamma4;

% state_variables = state_variables';
current_step_data = zeros(3,1);
current_step_data(1) = torque_error;
current_step_data(2) = current_learning_control_input;
current_step_data(3) = filtered_torque_error;
return

%% functions
% 位置跟踪
function desired_pos = pos_trajectory(current_time, state_start_time, pos_traj_mode, pos_des_1, pos_des_2)
state_time = current_time - state_start_time;
switch pos_traj_mode
    case 1
        phase_time = mod(state_time, 0.5);
        switch mod(ceil(state_time/0.5), 2)
            case 0
                desired_pos= -100 - phase_time*50;
            case 1
                desired_pos = 100 + phase_time*10;
            otherwise
                desired_pos = 0;
        end
    case 2
        if state_time < 2
            desired_pos = 0;
        elseif state_time < 7
            desired_pos = pos_des_1;
        else
            desired_pos = pos_des_2;
        end
    otherwise
        desired_pos = 0;
        
end


return
%%

%define desired trajectory 定义期望力矩曲线 
function torque = torque_curve(current_time, state_start_time, ...
    current_state, curve_id,...
    desired_torque_mag,...
    last_stride_time,  HLCParam, ankle_pos, xinit, K_curve, CusHLCInputs,oo_dtau_offset)


%State definitions
idle_state	=	0;
calibration_state	=   1;
stance_state   =   2;
swing_state     =   3;
step_state  =   4;


switch current_state
    case step_state % STEP
        switch curve_id
            case 4
                torque = 0;
            otherwise
                torque = desired_torque_mag;
        end
    case stance_state
        %         torque = -Kt*ankle_pos;
        switch curve_id
            case 1
                torque  = -K_curve*(ankle_pos-xinit);
                
            case 12
                
                %                 HLCParam = [1 10 20 50 30];
                torque = desired_torque_oo(HLCParam, current_time - state_start_time, last_stride_time);
                
            case 13
                %                 assert(HLCParamNo=6);
                %                 HLCParam = [1 10 20 50 30];
                torque = desired_torque_oo2(HLCParam, current_time - state_start_time, last_stride_time);
            case 14
                %                 assert(HLCParamNo=6);
                %                 HLCParam = [1 10 20 50 30];
                torque = desired_torque_oo3(HLCParam, current_time - state_start_time, last_stride_time);
            case 15
                %                 assert(HLCParamNo=6);
                %                 HLCParam = [1 10 20 50 30];
                torque = desired_torque_oo4(HLCParam, current_time - state_start_time, last_stride_time,oo_dtau_offset);
            
            case 16
                % 根据用户输入四参数CusHLCInputs生成期望力矩曲线
                torque = desired_torque_cus(current_time - state_start_time, last_stride_time, CusHLCInputs, oo_dtau_offset);
            otherwise
                torque = 0;
        end
    case swing_state
        switch curve_id
            case 4
                torque = 0;
            otherwise
                torque = 0;
        end
    otherwise
        torque = 0;
end
return






function torque = desired_torque_oo(params, current_stride_time, prev_stride_time)
i = length(params);
t = current_stride_time;

% distribute points from 0 - 25% 1/5, 25% to 45% 2/5 and 45% to 60% 2/5

m = floor(i*1/5);
n = floor(i*2/5);
k = i-m-n;


t_ankor = zeros(i+2, 1);
for j = 1:1:i
    if j<=m
        t_ankor(j+1) =  prev_stride_time*0.25/(m+1)*j;
        
    elseif j<=n
        t_ankor(j+1) = prev_stride_time*(0.25+0.2/(n+1)*(j-m));
    else
        t_ankor(j+1) = prev_stride_time*(0.45+0.15/(k+1)*(j-n-m));
    end;
end;
t_ankor(i+2)=prev_stride_time*0.6;
if iscolumn(params)
    allparams = params';
else
    allparams = params;
end;

tau_ankor = [0 allparams 0];

if current_stride_time <prev_stride_time*0.6
    torque  = cubicspline(t_ankor, tau_ankor, current_stride_time);
else
    torque = 0;
end;

torque = max(0, torque);

return;


function X = tridiag(L,D,U,B)
% X = tridiag(L,D,U,B)
% Solution of a tridiagonal linear system (LDU)X = B.
% It is assumed that D and B have dimension n,
% and that L and U have dimension n-1;
% L sub diagonal, input.
% D diagonal vector, input.
% U super diagonal, input.
% B right hand side vector, input.
% X solution vector, output.
n = length(B);
for k = 2:n,
    mult = L(k-1)/D(k-1);
    D(k) = D(k) - mult*U(k-1);
    B(k) = B(k) - mult*B(k-1); %forward substitution
end
X = zeros(n,1);
X(n) = B(n)/D(n);
for k = (n-1):-1:1,
    X(k) = (B(k) - U(k)*X(k+1))/D(k); %backward subtitution
end
return;

function u = cubicspline(x, y, t)
n=length(x);

h = zeros(1,n-1);
delta = zeros(1,n-1);
for i=1:n-1,
    
    h(i)=x(i+1)-x(i); delta(i)= (y(i+1)-y(i))/h(i);
    
end

%Construct the Tridiagonal System

hp=h(2:n-1); hm=h(1:n-2);
deltap=delta(2:n-1); deltam=delta(1:n-2);
U=[1,hm]; L=[hp,1]; D=2*[1,hp+hm,1];
B=3*[delta(1), hp.*deltam+hm.*deltap,delta(n-1)];
dy = tridiag(L,D,U,B);

%this is just the Cubic Hermite Graphing Code


if t>=x(n)
    u = 0;
else
    k = 1;
    for i=1:n-1,
        if t>=x(i) && t<x(i+1)
            k = i;
        end;
    end;
    
    
    a=delta(k);
    b=(a-dy(k))/h(k); c=(dy(k+1)-a)/h(k); d=(c-b)/h(k);
    u=y(k)+(t-x(k)).*(dy(k)+(t-x(k)).*(b+(t-x(k+1)).*d));
    
end
return;


function torque = desired_torque_oo2(params, current_stride_time, prev_stride_time)
%parameter size 6

t_ankor = [params(1) params(1)*0.67+params(4)*0.33 params(1)*0.33+params(4)*0.67  params(4) params(6)]/100*prev_stride_time;

tau_ankor = [0 params(2)*params(5)/100 params(3)*params(5)/100 params(5) 0];
% t_ankor=[0 t_ankor 0.8*prev_stride_time;];
% tau_ankor = [0 tau_ankor 0];

if (current_stride_time < t_ankor(1) || current_stride_time>t_ankor(end))
    torque = 0;
else
    %     torque  = mycubicspline(t_ankor, tau_ankor, 3, current_stride_time);
    torque  = mycubicspline(t_ankor, tau_ankor, 4, current_stride_time);
end;


function torque = desired_torque_oo3(params, current_stride_time, prev_stride_time)
%parameter size 6

t_ankor = [params(1) params(1)*0.67+params(4)*0.33 params(1)*0.33+params(4)*0.67  params(4) params(6)]/100*prev_stride_time;

tau_ankor = [0 params(2)*params(5)/100 params(3)*params(5)/100 params(5) 0];
% t_ankor=[0 t_ankor 0.8*prev_stride_time;];
% tau_ankor = [0 tau_ankor 0];

if (current_stride_time < t_ankor(1) || current_stride_time>t_ankor(end))
    torque = 0;
else
    %     torque  = mycubicspline(t_ankor, tau_ankor, 3, current_stride_time);
    torque  = interp1q(t_ankor', tau_ankor', current_stride_time);
end;

function torque = desired_torque_oo4(params, current_stride_time, prev_stride_time,oo_dtau_offset)
%parameter size 4

t_ankor = [params(2)/2-params(3) params(2)/2 params(2)/2+params(4)/2]/100*prev_stride_time;

tau_ankor = [0 params(1) 0];
% t_ankor=[0 t_ankor 0.8*prev_stride_time;];
% tau_ankor = [0 tau_ankor 0];

if (current_stride_time < t_ankor(1) || current_stride_time>t_ankor(end))
    torque = 0;
else
    torque  = mycubicspline(t_ankor, tau_ankor, 2, current_stride_time);
    %     torque  = interp1q(t_ankor', tau_ankor', current_stride_time);
end;
torque = torque + oo_dtau_offset;

tt = params(2)/2-params(3);
if current_stride_time<(prev_stride_time*tt/100)
    torque = current_stride_time/(prev_stride_time*tt/100)*oo_dtau_offset;
end;
tt2 =params(2)/2+params(4)/2;
if tt2<65
    if current_stride_time>(prev_stride_time*tt2/100)
        torque = (prev_stride_time*0.65-current_stride_time)/(prev_stride_time*(0.65-tt2/100))*oo_dtau_offset;
    end;
end;

if current_stride_time>(prev_stride_time*0.65)
torque =0;
end;


function torque = desired_torque_cus(current_stride_time, prev_stride_time, CusHLCInputs,oo_dtau_offset)
%parameter size 4
peakTorque = CusHLCInputs(1);
peakTime = CusHLCInputs(2);
riseTime = CusHLCInputs(3);
dropTime = CusHLCInputs(4);



t_ankor = [peakTime-riseTime peakTime peakTime+dropTime]/100*prev_stride_time;

tau_ankor = [0 peakTorque 0];
% t_ankor=[0 t_ankor 0.8*prev_stride_time;];
% tau_ankor = [0 tau_ankor 0];

if (current_stride_time < t_ankor(1) || current_stride_time>t_ankor(end))
    torque = 0;
else
    torque  = mycubicspline(t_ankor, tau_ankor, 2, current_stride_time);
    %     torque  = interp1q(t_ankor', tau_ankor', current_stride_time);
end;

torque = torque + oo_dtau_offset;

tt =peakTime-riseTime;
if current_stride_time<(prev_stride_time*tt/100)
torque = current_stride_time/(prev_stride_time*tt/100)*oo_dtau_offset;
end;
tt2 =peakTime+dropTime;
if tt2<65
    if current_stride_time>(prev_stride_time*tt2/100)
        torque = (prev_stride_time*0.65-current_stride_time)/(prev_stride_time*(0.65-tt2/100))*oo_dtau_offset;
    end;
end;
if current_stride_time>(prev_stride_time*0.65)
torque =0;
end;


function u = mycubicspline(x, y, ip, t)
% x and y are the coordinates of the ankor nodes
% ip is the index of peak/valley point
n=length(x);

h = zeros(1,n-1);
delta = zeros(1,n-1);
for i=1:n-1,
    
    h(i)=x(i+1)-x(i); delta(i)= (y(i+1)-y(i))/h(i);
    
end

%Construct the Tridiagonal System

hp=h(2:n-1); hm=h(1:n-2);
deltap=delta(2:n-1); deltam=delta(1:n-2);
U=[1,hm]; L=[hp,1]; D=2*[1,hp+hm,1];
B=3*[delta(1), hp.*deltam+hm.*deltap,delta(n-1)];
% L
% D
% U
% B
% dy = tridiag(L,D,U,B)
dy = tridiag2(L,D,U,B,ip);

%this is just the Cubic Hermite Graphing Code


if t>=x(n)
    u = 0;
elseif t<=x(1)
    u = 0;
else
    k = 1;
    for i=1:n-1
        if t>=x(i) && t<x(i+1)
            k = i;
        end
    end
    
    
    a=delta(k);
    b=(a-dy(k))/h(k); c=(dy(k+1)-a)/h(k); d=(c-b)/h(k);
    u=y(k)+(t-x(k)).*(dy(k)+(t-x(k)).*(b+(t-x(k+1)).*d));
    
end
return;

function X = tridiag2(L,D,U,B,ip)
% X = tridiag(L,D,U,B)
% Solution of a tridiagonal linear system (LDU)X = B.
% It is assumed that D and B have dimension n,
% and that L and U have dimension n-1;
% L sub diagonal, input.
% D diagonal vector, input.
% U super diagonal, input.
% B right hand side vector, input.
% X solution vector, output.
n = length(B);
% for k = 2:n,
%     mult = L(k-1)/D(k-1);
%     D(k) = D(k) - mult*U(k-1);
%     B(k) = B(k) - mult*B(k-1); %forward substitution
% end
%
% X = zeros(n,1);
%
% % D(end, :)  = zeros(size(D(end,:)));
% % D(end, ip) = 1;
% % B(end) = 0;
%
% X(n) = B(n)/D(n);
%
% for k = (n-1):-1:1,
%     X(k) = (B(k) - U(k)*X(k+1))/D(k); %backward subtitution
% end
UU = [[zeros(n-1, 1) diag(U)]; zeros(1, n)];
LL = [zeros(1, n); [diag(L) zeros(n-1, 1)]];
DD = diag(D);
DD = UU+LL+DD;
B(ip) = 0;
DD(ip, :)  = zeros(size(DD(ip,:)));
DD(ip, ip) = 1;
B(1) = 0;
DD(1, :)  = zeros(size(DD(ip,:)));
DD(1, 1) = 1;

% B(1) = 0;
% DD(1, :)  = zeros(size(DD(1,:)));
% DD(1, 1) = 1;

X= DD\B';
return;
